simulink model "sdl_testbed"  (R2022b)
settings: Solver=VariableStepAuto  StartTime=0.0  StopTime=5  RelTol=1e-3  AbsTol=1e-3  EnableMultiTasking=on
PreLoadFcn:
  | MFormulaCoeff.DryTarmac = [10 1.9 1 0.97];
  | MFormulaCoeff.WetTarmac = [12 2.3 0.82 1];
  | MFormulaCoeff.Snow         = [5 2 0.3 1];
  | MFormulaCoeff.Ice            = [4 2 0.1 1];
libraries: sdl_lib x22, nesl_utility x9, fl_ps_legacy_lib x5, fl_lib x4, simulink x1
(part 2 of 3)

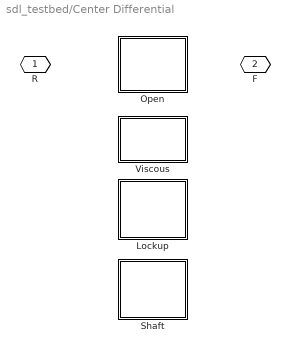
== system sdl_testbed/Center Differential ==
  Lockup : Subsystem  Tag=PublishSubsystem  VariantControl=Lockup
      mask Display:
      | %patch([0;227.23643342033;227.23643342033;0;0;0.472425017505884;0.472425017505884;226.764008402824;226.764008402824;0.472425017505884;0], [170.545431319624;170.545431319624;0;0;170.545431319624;170.073006302118;0.472425017505884;0.472425017505884;170.073006302118;170.073006302118;170.545431319624], [1;1;1])
      | plot([0;227.23643342033;227.23643342033;0;0;0.472425017505884;0.472425017505884;226.764008402824;226.764008402824;0.472425017505884;0], [170.545431319624;170.545431319624;0;0;170.545431319624;170.073006302118;0.472425017505884;0.472425017505884;170.073006302118;170.073006302118;170.545431319624])
      | plot([136.294617550448;187.000220911577], [85.2727156598121;85.2727156598121])
      | plot([40.236212508752942;90.9418158698827], [85.2727156598121;85.2727156598121])
      | patch([130.625517340377;136.294617550448;136.294617550448;130.625517340377;130.625517340377], [141.963717760518;141.963717760518;28.581713559106;28.581713559106;141.963717760518], [0;0;0])
      | plot([130.625517340377;136.294617550448;136.294617550448;130.625517340377;130.625517340377], [141.963717760518;141.963717760518;28.581713559106;28.581713559106;141.963717760518])
      | patch([90.9418158698827;96.6109160799533;96.6109160799533;90.9418158698827;90.9418158698827], [141.963717760518;141.963717760518;28.581713559106;28.581713559106;141.963717760518], [0;0;0])
      | plot([90.9418158698827;96.6109160799533;96.6109160799533;90.9418158698827;90.9418158698827], [141.963717760518;141.963717760518;28.581713559106;28.581713559106;141.963717760518])
      | patch([110.78366660513;116.4527668152;116.4527668152;110.78366660513;110.78366660513], [141.963717760518;141.963717760518;28.581713559106;28.581713559106;141.963717760518], [0;0;0])
      | plot([110.78366660513;116.4527668152;116.4527668152;110.78366660513;110.78366660513], [141.963717760518;141.963717760518;28.581713559106;28.581713559106;141.963717760518])
  Open : Subsystem  VariantControl=Open
      mask Display:
      | %patch([0;227.23643342033;227.23643342033;0;0;0.472425017505884;0.472425017505884;226.764008402824;226.764008402824;0.472425017505884;0], [170.545431319624;170.545431319624;0;0;170.545431319624;170.073006302118;0.472425017505884;0.472425017505884;170.073006302118;170.073006302118;170.545431319624], [1;1;1])
      | plot([0;227.23643342033;227.23643342033;0;0;0.472425017505884;0.472425017505884;226.764008402824;226.764008402824;0.472425017505884;0], [170.545431319624;170.545431319624;0;0;170.545431319624;170.073006302118;0.472425017505884;0.472425017505884;170.073006302118;170.073006302118;170.545431319624])
      | plot([136.294617550448;187.000220911577], [85.2727156598121;85.2727156598121])
      | plot([40.236212508752942;90.9418158698827], [85.2727156598121;85.2727156598121])
  Shaft : Subsystem  VariantControl=Shaft
      mask Display:
      | %patch([0;227.23643342033;227.23643342033;0;0;0.472425017505884;0.472425017505884;226.764008402824;226.764008402824;0.472425017505884;0], [170.545431319624;170.545431319624;0;0;170.545431319624;170.073006302118;0.472425017505884;0.472425017505884;170.073006302118;170.073006302118;170.545431319624], [1;1;1])
      | plot([0;227.23643342033;227.23643342033;0;0;0.472425017505884;0.472425017505884;226.764008402824;226.764008402824;0.472425017505884;0], [170.545431319624;170.545431319624;0;0;170.545431319624;170.073006302118;0.472425017505884;0.472425017505884;170.073006302118;170.073006302118;170.545431319624])
      | patch([40.236212508752942;40.236212508752942;187.9418158698827;187.9418158698827;40.236212508752942], [80.2727156598121;90.2727156598121;90.2727156598121;80.2727156598121;80.2727156598121])
  Viscous : Subsystem  VariantControl=Viscous
      mask Display:
      | %patch([-40;267.23643342033;267.23643342033;-40;-40;-40.472425017505884;-40.472425017505884;266.764008402824;266.764008402824;-40.472425017505884;-40], [170.545431319624;170.545431319624;0;0;170.545431319624;170.073006302118;0.472425017505884;0.472425017505884;170.073006302118;170.073006302118;170.545431319624], [1;1;1])
      | plot([-40;267.23643342033;267.23643342033;-40;-40;-40.472425017505884;-40.472425017505884;266.764008402824;266.764008402824;-40.472425017505884;-40], [170.545431319624;170.545431319624;0;0;170.545431319624;170.073006302118;0.472425017505884;0.472425017505884;170.073006302118;170.073006302118;170.545431319624])
      | plot([15.236212508752942;113.618216710165], [85.2727156598121;85.2727156598121])
      | plot([71.0999651346356;156.136468285695;156.136468285695;71.0999651346356], [144.798267865554;122.121867025271;48.4235642943531;25.7471634540707])
      | plot([156.136468285695;212.000220911577], [85.2727156598121;85.2727156598121])
      | plot([113.618216710165;113.618216710165], [123.570637078956;46.4078842196614])
      | plot([113.618216710165;113.618216710165], [46.4078842196614;45.5890141893178])
      | plot([96.6109160799533;136.294617550448], [42.7544640842825;51.2581143993884])
      | plot([93.776365974918;133.460067445412], [127.790967235342;119.287316920236])
  R : PMIOPort  Side=Left
  F : PMIOPort  Port=2  Side=Right

== system sdl_testbed/Front Differential ==
  Open : Subsystem  VariantControl=Open
      mask Display:
      | plot([73.6983027309179;73.6983027309179], [209.756707772613;130.389304831624])
      | plot([73.6983027309179;39.6837014704943], [170.073006302118;170.073006302118])
      | plot([62.3601023107767;85.0365031510592], [221.094908192754;198.418507352471])
      | plot([85.0365031510592;62.3601023107767], [141.727505251765;119.051104411483])
      | plot([102.043803781271;119.051104411483;119.051104411483;198.418507352471;198.418507352471], [181.41120672226;181.41120672226;260.778609663248;260.778609663248;277.78591029346])
      | plot([164.403906092048;255.109509453177], [226.764008402824;226.764008402824])
      | plot([153.065705671906;153.065705671906], [215.425807982683;124.720204621553])
      | plot([209.756707772613;209.756707772613], [317.469611763954;226.764008402824])
      | plot([187.08030693233;198.418507352471], [277.78591029346;277.78591029346])
      | plot([141.727505251765;164.403906092048], [226.764008402824;204.087607562542])
      | plot([175.742106512189;153.065705671906], [124.720204621553;102.043803781271])
      | plot([153.065705671906;175.742106512189], [238.102208822966;215.425807982683])
      | plot([209.756707772613;209.756707772613], [113.382004201412;22.6764008402824])
      | plot([164.403906092048;141.727505251765], [136.058405041695;113.382004201412])
      | plot([243.771309033036;266.447709873319], [124.720204621553;102.043803781271])
      | plot([266.447709873319;243.771309033036], [238.102208822966;215.425807982683])
      | plot([164.403906092048;255.109509453177], [113.382004201412;113.382004201412])
      | plot([187.08030693233;198.418507352471;198.418507352471;119.051104411483;119.051104411483;102.043803781271;102.043803781271], [62.3601023107767;62.3601023107767;79.3674029409885;79.3674029409885;158.734805881977;158.734805881977;147.396605461836])
      | plot([102.043803781271;153.065705671906], [170.073006302118;170.073006302118])
      | plot([102.043803781271;102.043803781271], [181.41120672226;192.749407142401])
      | plot([96.3747035712004;73.6983027309179], [130.389304831624;107.712903991342])
      | plot([85.0365031510592;119.051104411483], [119.051104411483;119.051104411483])
      | plot([-20;-20;360.146012604237;360.146012604237;-20], [360.146012604237;-20;-20;360.146012604237;360.146012604237])
  Torsen : Subsystem  VariantControl=Torsen
      mask Display:
      | plot([73.6983027309179;73.6983027309179], [209.756707772613;130.389304831624])
      | plot([73.6983027309179;39.6837014704943], [170.073006302118;170.073006302118])
      | 
      | % Planet Gear
      | plot([164.403906092048;255.109509453177;255.109509453177;164.403906092048;164.403906092048], [226.764008402824;226.764008402824;226.764008402824-50;226.764008402824-50;226.764008402824])
      | plot([164.403906092048;255.109509453177;255.109509453177;164.403906092048;164.403906092048], [113.382004201412;113.382004201412;113.382004201412+50;113.382004201412+50;113.382004201412])
      | plot([164.403906092048  ;164.403906092048+50]+ 0, [176.764008402824   ;176.764008402824+50])
      | plot([164.403906092048  ;164.403906092048+50]+20, [176.764008402824   ;176.764008402824+50])
      | plot([164.403906092048  ;164.403906092048+50]+40, [176.764008402824   ;176.764008402824+50])
      | plot([164.403906092048  ;164.403906092048+30]+60, [176.764008402824   ;176.764008402824+30])
      | plot([164.403906092048+20;164.403906092048+50]-20,[176.764008402824+20;176.764008402824+50])
      | 
      | plot([164.403906092048  ;164.403906092048+50]+ 0, [113.382004201412   ;113.382004201412+50])
      | plot([164.403906092048  ;164.403906092048+50]+20, [113.382004201412   ;113.382004201412+50])
      | plot([164.403906092048  ;164.403906092048+50]+40, [113.382004201412   ;113.382004201412+50])
      | plot([164.403906092048  ;164.403906092048+30]+60, [113.382004201412   ;113.382004201412+30])
      | plot([164.403906092048+20;164.403906092048+50]-20,[113.382004201412+20;113.382004201412+50])
      | 
      | plot(sin(0:0.1:6*pi)*20+140,cos(0:0.1:6*pi)*25+138);
      | plot(sin(0:0.1:6*pi)*25+140,cos(0:0.1:6*pi)*32+138);
      | plot(sin(0:0.1:6*pi)*20+140,cos(0:0.1:6*pi)*25+203);
      | plot(sin(0:0.1:6*pi)*25+140,cos(0:0.1:6*pi)*32+203);
      | 
      | 
      | plot([209.756707772613;209.756707772613], [317.469611763954;226.764008402824])
      | plot([209.756707772613;209.756707772613], [113.382004201412;22.6764008402824])
      | 
      | % Housing
      | plot([102.043803781271;119.051104411483;119.051104411483;198.418507352471;198.418507352471]-28, [181.41120672226;181.41120672226;260.778609663248;260.778609663248;277.78591029346])
      | plot([102.043803781271;102.043803781271]-28, [181.41120672226;192.749407142401])
      | plot([187.08030693233;198.418507352471]-28, [277.78591029346;277.78591029346])
      | plot([187.08030693233;198.418507352471;198.418507352471;119.051104411483;119.051104411483;102.043803781271;102.043803781271]-28, [62.3601023107767;62.3601023107767;79.3674029409885;79.3674029409885;158.734805881977;158.734805881977;147.396605461836])
      | 
      | plot([-20;-20;330.146012604237;330.146012604237;-20], [370.146012604237;-20;-20;370.146012604237;370.146012604237])
  D : PMIOPort  Side=Left
  S1 : PMIOPort  Port=2  Side=Right
  S2 : PMIOPort  Port=3  Side=Right

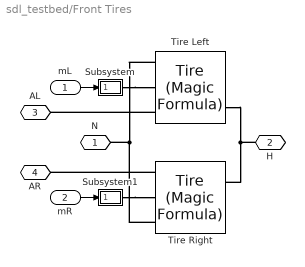
== system sdl_testbed/Front Tires ==
  mL : Inport
  mR : Inport  Port=2
  Subsystem : Subsystem
      mask Display: disp('PS')
  Subsystem1 : Subsystem
      mask Display: disp('PS')
  Tire Left : sdl_lib/Tires & Vehicles/Tire (Magic Formula)  parameterization=4  F_z1=3e+3 N  F_x1=3.5e+3 N  kappa1=10  B_m=10  C_m=1.9  D_m=1  E_m=0.97  fz0=4e+3 N  p_Cx=1.685  p_Dx=[ 1.21 -0.037 ]  p_Ex=[ 0.344 0.095 -0.02 0 ]  p_Kx=[ 21.51 -0.163 0.245 ]  p_Hx=[ -0.002 0.002 ]  p_Vx=[ 0 0 ]  r_e=0.3 m  model_compliance=0  stiffness=1e+6 N/m  damping=1000 N/(m/s)  model_inertia=1  inertia=1 kg*m^2  initial_velocity=0 rad/s  model_resistance=0  resistance_model=1  coeff=0.015  p_tire=250e3 Pa  alpha=-0.003  beta=0.97  coeff_a=84e-4  coeff_b=6.2e-4 s/m  coeff_c=1.6e-4 s^2/m^2  v_thr=1e-3 m/s  v_tr_thr=0.1 m/s
      settings: InternalSimscapePortConfiguration="{\"Bottom\":[],\"Left\":[{\"id\":\"N\",\"label\":\"N\",\"type\":\"input\"},{\"id\":\"M\",\"label\":\"M\",\"type\":\"input\"},{\"id\":\"A\",\"label\":\"A\",\"type\":\"foundation.mechanical.rotational.rotational\"}],\"Right\":[{\"id\":\"S\",\"label\":\"S\",\"type\":\"output\"},{\"id\":\"H\",\"label\":\"H\",\"type\":\"foundation.mechanical.translational.translational\"}],\"Top\":[]}"
  Tire Right : sdl_lib/Tires & Vehicles/Tire (Magic Formula)  parameterization=4  F_z1=3e+3 N  F_x1=3.5e+3 N  kappa1=10  B_m=10  C_m=1.9  D_m=1  E_m=0.97  fz0=4e+3 N  p_Cx=1.685  p_Dx=[ 1.21 -0.037 ]  p_Ex=[ 0.344 0.095 -0.02 0 ]  p_Kx=[ 21.51 -0.163 0.245 ]  p_Hx=[ -0.002 0.002 ]  p_Vx=[ 0 0 ]  r_e=0.3 m  model_compliance=0  stiffness=1e+6 N/m  damping=1000 N/(m/s)  model_inertia=1  inertia=1 kg*m^2  initial_velocity=0 rad/s  model_resistance=0  resistance_model=1  coeff=0.015  p_tire=250e3 Pa  alpha=-0.003  beta=0.97  coeff_a=84e-4  coeff_b=6.2e-4 s/m  coeff_c=1.6e-4 s^2/m^2  v_thr=1e-3 m/s  v_tr_thr=0.1 m/s
      settings: InternalSimscapePortConfiguration="{\"Bottom\":[],\"Left\":[{\"id\":\"N\",\"label\":\"N\",\"type\":\"input\"},{\"id\":\"M\",\"label\":\"M\",\"type\":\"input\"},{\"id\":\"A\",\"label\":\"A\",\"type\":\"foundation.mechanical.rotational.rotational\"}],\"Right\":[{\"id\":\"S\",\"label\":\"S\",\"type\":\"output\"},{\"id\":\"H\",\"label\":\"H\",\"type\":\"foundation.mechanical.translational.translational\"}],\"Top\":[]}"
  N : PMIOPort  Side=Right
  H : PMIOPort  Port=2  Side=Right
  AL : PMIOPort  Port=3  Side=Right
  AR : PMIOPort  Port=4  Side=Right
  wires:
  mR/1 -> Subsystem1/1(In1)
  mL/1 -> Subsystem/1(In1)
  connections:
  Subsystem/RConn1 -- Tire Left/LConn2
  Subsystem1/RConn1 -- Tire Right/LConn2
  Tire Right/LConn3 -- AR/RConn1
  Tire Left/LConn1 -- Tire Right/LConn1 -- N/RConn1
  Tire Left/RConn2 -- Tire Right/RConn2 -- H/RConn1
  Tire Left/LConn3 -- AL/RConn1

== system sdl_testbed/Rear Differential ==
  Open : Subsystem  Tag=PublishSubsystem  VariantControl=Open
      mask Display:
      | plot([73.6983027309179;73.6983027309179], [209.756707772613;130.389304831624])
      | plot([73.6983027309179;39.6837014704943], [170.073006302118;170.073006302118])
      | plot([62.3601023107767;85.0365031510592], [221.094908192754;198.418507352471])
      | plot([85.0365031510592;62.3601023107767], [141.727505251765;119.051104411483])
      | plot([102.043803781271;119.051104411483;119.051104411483;198.418507352471;198.418507352471], [181.41120672226;181.41120672226;260.778609663248;260.778609663248;277.78591029346])
      | plot([164.403906092048;255.109509453177], [226.764008402824;226.764008402824])
      | plot([153.065705671906;153.065705671906], [215.425807982683;124.720204621553])
      | plot([209.756707772613;209.756707772613], [317.469611763954;226.764008402824])
      | plot([187.08030693233;198.418507352471], [277.78591029346;277.78591029346])
      | plot([141.727505251765;164.403906092048], [226.764008402824;204.087607562542])
      | plot([175.742106512189;153.065705671906], [124.720204621553;102.043803781271])
      | plot([153.065705671906;175.742106512189], [238.102208822966;215.425807982683])
      | plot([209.756707772613;209.756707772613], [113.382004201412;22.6764008402824])
      | plot([164.403906092048;141.727505251765], [136.058405041695;113.382004201412])
      | plot([243.771309033036;266.447709873319], [124.720204621553;102.043803781271])
      | plot([266.447709873319;243.771309033036], [238.102208822966;215.425807982683])
      | plot([164.403906092048;255.109509453177], [113.382004201412;113.382004201412])
      | plot([187.08030693233;198.418507352471;198.418507352471;119.051104411483;119.051104411483;102.043803781271;102.043803781271], [62.3601023107767;62.3601023107767;79.3674029409885;79.3674029409885;158.734805881977;158.734805881977;147.396605461836])
      | plot([102.043803781271;153.065705671906], [170.073006302118;170.073006302118])
      | plot([102.043803781271;102.043803781271], [181.41120672226;192.749407142401])
      | plot([96.3747035712004;73.6983027309179], [130.389304831624;107.712903991342])
      | plot([85.0365031510592;119.051104411483], [119.051104411483;119.051104411483])
      | plot([-20;-20;360.146012604237;360.146012604237;-20], [360.146012604237;-20;-20;360.146012604237;360.146012604237])
  Torsen : Subsystem  Tag=PublishSubsystem  VariantControl=Torsen
      mask Display:
      | plot([73.6983027309179;73.6983027309179], [209.756707772613;130.389304831624])
      | plot([73.6983027309179;39.6837014704943], [170.073006302118;170.073006302118])
      | 
      | % Planet Gear
      | plot([164.403906092048;255.109509453177;255.109509453177;164.403906092048;164.403906092048], [226.764008402824;226.764008402824;226.764008402824-50;226.764008402824-50;226.764008402824])
      | plot([164.403906092048;255.109509453177;255.109509453177;164.403906092048;164.403906092048], [113.382004201412;113.382004201412;113.382004201412+50;113.382004201412+50;113.382004201412])
      | plot([164.403906092048  ;164.403906092048+50]+ 0, [176.764008402824   ;176.764008402824+50])
      | plot([164.403906092048  ;164.403906092048+50]+20, [176.764008402824   ;176.764008402824+50])
      | plot([164.403906092048  ;164.403906092048+50]+40, [176.764008402824   ;176.764008402824+50])
      | plot([164.403906092048  ;164.403906092048+30]+60, [176.764008402824   ;176.764008402824+30])
      | plot([164.403906092048+20;164.403906092048+50]-20,[176.764008402824+20;176.764008402824+50])
      | 
      | plot([164.403906092048  ;164.403906092048+50]+ 0, [113.382004201412   ;113.382004201412+50])
      | plot([164.403906092048  ;164.403906092048+50]+20, [113.382004201412   ;113.382004201412+50])
      | plot([164.403906092048  ;164.403906092048+50]+40, [113.382004201412   ;113.382004201412+50])
      | plot([164.403906092048  ;164.403906092048+30]+60, [113.382004201412   ;113.382004201412+30])
      | plot([164.403906092048+20;164.403906092048+50]-20,[113.382004201412+20;113.382004201412+50])
      | 
      | plot(sin(0:0.1:6*pi)*20+140,cos(0:0.1:6*pi)*25+138);
      | plot(sin(0:0.1:6*pi)*25+140,cos(0:0.1:6*pi)*32+138);
      | plot(sin(0:0.1:6*pi)*20+140,cos(0:0.1:6*pi)*25+203);
      | plot(sin(0:0.1:6*pi)*25+140,cos(0:0.1:6*pi)*32+203);
      | 
      | 
      | plot([209.756707772613;209.756707772613], [317.469611763954;226.764008402824])
      | plot([209.756707772613;209.756707772613], [113.382004201412;22.6764008402824])
      | 
      | % Housing
      | plot([102.043803781271;119.051104411483;119.051104411483;198.418507352471;198.418507352471]-28, [181.41120672226;181.41120672226;260.778609663248;260.778609663248;277.78591029346])
      | plot([102.043803781271;102.043803781271]-28, [181.41120672226;192.749407142401])
      | plot([187.08030693233;198.418507352471]-28, [277.78591029346;277.78591029346])
      | plot([187.08030693233;198.418507352471;198.418507352471;119.051104411483;119.051104411483;102.043803781271;102.043803781271]-28, [62.3601023107767;62.3601023107767;79.3674029409885;79.3674029409885;158.734805881977;158.734805881977;147.396605461836])
      | 
      | plot([-20;-20;330.146012604237;330.146012604237;-20], [370.146012604237;-20;-20;370.146012604237;370.146012604237])
  D : PMIOPort  Side=Left
  S1 : PMIOPort  Port=2  Side=Right
  S2 : PMIOPort  Port=3  Side=Right

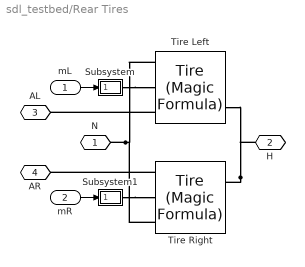
== system sdl_testbed/Rear Tires ==
  mL : Inport
  mR : Inport  Port=2
  Subsystem : Subsystem
      mask Display: disp('PS')
  Subsystem1 : Subsystem
      mask Display: disp('PS')
  Tire Left : sdl_lib/Tires & Vehicles/Tire (Magic Formula)  parameterization=4  F_z1=3e+3 N  F_x1=3.5e+3 N  kappa1=10  B_m=10  C_m=1.9  D_m=1  E_m=0.97  fz0=4e+3 N  p_Cx=1.685  p_Dx=[ 1.21 -0.037 ]  p_Ex=[ 0.344 0.095 -0.02 0 ]  p_Kx=[ 21.51 -0.163 0.245 ]  p_Hx=[ -0.002 0.002 ]  p_Vx=[ 0 0 ]  r_e=0.3 m  model_compliance=0  stiffness=1e+6 N/m  damping=1000 N/(m/s)  model_inertia=1  inertia=1 kg*m^2  initial_velocity=0 rad/s  model_resistance=0  resistance_model=1  coeff=0.015  p_tire=250e3 Pa  alpha=-0.003  beta=0.97  coeff_a=84e-4  coeff_b=6.2e-4 s/m  coeff_c=1.6e-4 s^2/m^2  v_thr=1e-3 m/s  v_tr_thr=0.1 m/s
      settings: InternalSimscapePortConfiguration="{\"Bottom\":[],\"Left\":[{\"id\":\"N\",\"label\":\"N\",\"type\":\"input\"},{\"id\":\"M\",\"label\":\"M\",\"type\":\"input\"},{\"id\":\"A\",\"label\":\"A\",\"type\":\"foundation.mechanical.rotational.rotational\"}],\"Right\":[{\"id\":\"S\",\"label\":\"S\",\"type\":\"output\"},{\"id\":\"H\",\"label\":\"H\",\"type\":\"foundation.mechanical.translational.translational\"}],\"Top\":[]}"
  Tire Right : sdl_lib/Tires & Vehicles/Tire (Magic Formula)  parameterization=4  F_z1=3e+3 N  F_x1=3.5e+3 N  kappa1=10  B_m=10  C_m=1.9  D_m=1  E_m=0.97  fz0=4e+3 N  p_Cx=1.685  p_Dx=[ 1.21 -0.037 ]  p_Ex=[ 0.344 0.095 -0.02 0 ]  p_Kx=[ 21.51 -0.163 0.245 ]  p_Hx=[ -0.002 0.002 ]  p_Vx=[ 0 0 ]  r_e=0.3 m  model_compliance=0  stiffness=1e+6 N/m  damping=1000 N/(m/s)  model_inertia=1  inertia=1 kg*m^2  initial_velocity=0 rad/s  model_resistance=0  resistance_model=1  coeff=0.015  p_tire=250e3 Pa  alpha=-0.003  beta=0.97  coeff_a=84e-4  coeff_b=6.2e-4 s/m  coeff_c=1.6e-4 s^2/m^2  v_thr=1e-3 m/s  v_tr_thr=0.1 m/s
      settings: InternalSimscapePortConfiguration="{\"Bottom\":[],\"Left\":[{\"id\":\"N\",\"label\":\"N\",\"type\":\"input\"},{\"id\":\"M\",\"label\":\"M\",\"type\":\"input\"},{\"id\":\"A\",\"label\":\"A\",\"type\":\"foundation.mechanical.rotational.rotational\"}],\"Right\":[{\"id\":\"S\",\"label\":\"S\",\"type\":\"output\"},{\"id\":\"H\",\"label\":\"H\",\"type\":\"foundation.mechanical.translational.translational\"}],\"Top\":[]}"
  N : PMIOPort  Side=Right
  H : PMIOPort  Port=2  Side=Right
  AL : PMIOPort  Port=3  Side=Right
  AR : PMIOPort  Port=4  Side=Right
  wires:
  mL/1 -> Subsystem/1(In1)
  mR/1 -> Subsystem1/1(In1)
  connections:
  Tire Left/LConn3 -- AL/RConn1
  Tire Right/RConn2 -- H/RConn1 -- Tire Left/RConn2
  N/RConn1 -- Tire Right/LConn1 -- Tire Left/LConn1
  Tire Right/LConn3 -- AR/RConn1
  Subsystem1/RConn1 -- Tire Right/LConn2
  Subsystem/RConn1 -- Tire Left/LConn2

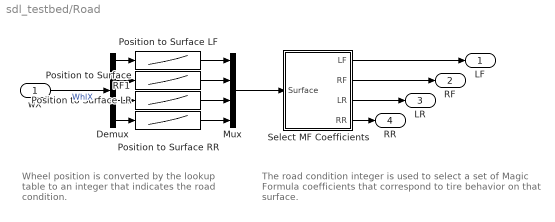
== system sdl_testbed/Road ==
  note: Wheel position is converted by the
      | lookup table to an integer
      | that indicates the road condition.
  note: The road condition integer is used to select
      | a set of Magic Formula coefficients
      | that correspond to tire behavior on that surface.
  wX : Inport
  Demux : Demux
  Mux : Mux
  Position to Surface LF : Lookup_n-D  NumberOfTableDimensions=1  LookupTableObject=''  BreakpointsForDimension1=surface_xpos  BeginIndexSearchUsingPreviousIndexResult=on  Table=surface_LF  InterpMethod=Flat  InternalRulePriority=Speed  RndMeth=Simplest
  Position to Surface LR : Lookup_n-D  NumberOfTableDimensions=1  LookupTableObject=''  BreakpointsForDimension1=surface_xpos  BeginIndexSearchUsingPreviousIndexResult=on  Table=surface_LR  InterpMethod=Flat  InternalRulePriority=Speed  RndMeth=Simplest
  Position to Surface RF1 : Lookup_n-D  NumberOfTableDimensions=1  LookupTableObject=''  BreakpointsForDimension1=surface_xpos  BeginIndexSearchUsingPreviousIndexResult=on  Table=surface_RF  InterpMethod=Flat  InternalRulePriority=Speed  RndMeth=Simplest
  Position to Surface RR : Lookup_n-D  NumberOfTableDimensions=1  LookupTableObject=''  BreakpointsForDimension1=surface_xpos  BeginIndexSearchUsingPreviousIndexResult=on  Table=surface_RR  InterpMethod=Flat  InternalRulePriority=Speed  RndMeth=Simplest
  Select MF Coefficients : Subsystem
  LF : Outport  VectorParamsAs1DForOutWhenUnconnected=off
  RF : Outport  Port=2  VectorParamsAs1DForOutWhenUnconnected=off
  LR : Outport  Port=3  VectorParamsAs1DForOutWhenUnconnected=off
  RR : Outport  Port=4  VectorParamsAs1DForOutWhenUnconnected=off
  wires:
  Select MF Coefficients/3(LR) -> LR/1
  Select MF Coefficients/4(RR) -> RR/1
  Select MF Coefficients/1(LF) -> LF/1
  Select MF Coefficients/2(RF) -> RF/1
  wX/1 -> Demux/1  "WhlX"
  Mux/1 -> Select MF Coefficients/1(Surface)
  Demux/1 -> Position to Surface LF/1
  Position to Surface LF/1 -> Mux/1
  Position to Surface RR/1 -> Mux/4
  Demux/4 -> Position to Surface RR/1
  Demux/2 -> Position to Surface RF1/1
  Position to Surface RF1/1 -> Mux/2
  Position to Surface LR/1 -> Mux/3
  Demux/3 -> Position to Surface LR/1

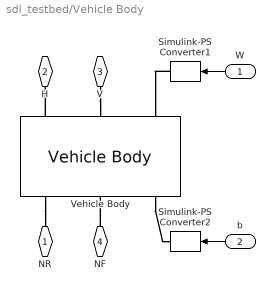
== system sdl_testbed/Vehicle Body ==
  W : Inport
  b : Inport  Port=2
  Simulink-PS Converter1 : nesl_utility/Simulink-PS Converter  PhysicalDomain=network_engine_domain  SubClassName=ps_input  LeftPortType=input  RightPortType=output  PseudoPeriodic=off  Frequencies=[]  NoiseDistribution=none  NoiseParameters=[]  Unit=m/s  AffineConversion=off  FilteringAndDerivatives=zero  SimscapeFilterOrder=1  InputFilterTimeConstant=.001  UdotUserProvided=1
  Simulink-PS Converter2 : nesl_utility/Simulink-PS Converter  PhysicalDomain=network_engine_domain  SubClassName=ps_input  LeftPortType=input  RightPortType=output  PseudoPeriodic=off  Frequencies=[]  NoiseDistribution=none  NoiseParameters=[]  Unit=deg  AffineConversion=off  FilteringAndDerivatives=zero  SimscapeFilterOrder=1  InputFilterTimeConstant=.001  UdotUserProvided=1
  Vehicle Body : sdl_lib/Tires & Vehicles/Vehicle Body  mass=1000 kg  n_w=2  x_f=1.4 m  x_r=1.6 m  y_c=0.5 m  mass_var=simscape.enum.onoff.off  g=9.81 m/s^2  liftoff_warning=0  area=3 m^2  Cd=0.4  rho=1.18 kg/m^3  model_pitch=0  inertia=4000 kg*m^2  suspension_model=1  k_f=1e4 N/m  b_f=1e4 N/(m/s)  k_r=1e4 N/m  b_r=1e4 N/(m/s)  k_f_TLU=[-2000, -1000, 0, 1000, 2000] N  x_f_TLU=[-.4, -.2, 0, .2, .4] m  b_f_TLU=[-200, -100, 0, 100, 200] N  v_f_TLU=[-4, -2, 0, 2, 4] m/s  k_r_TLU=[-2000, -1000, 0, 1000, 2000] N  x_r_TLU=[-.4, -.2, 0, .2, .4] m  b_r_TLU=[-200, -100, 0, 100, 200] N  v_r_TLU=[-4, -2, 0, 2, 4] m/s  interp_method=simscape.enum.interpolation.linear  extrap_method=simscape.enum.extrapolation.linear  model_hardstop=0  upper_bound_f=.25 m  lower_bound_f=-.25 m  stop_k_f=1e6 N/m  stop_b_f=150 N/(m/s)  upper_bound_r=.25 m  lower_bound_r=-.25 m  stop_k_r=1e6 N/m  stop_b_r=150 N/(m/s)  initial_pitch=0 rad  initial_pitch_rate=0 rad/s  v_specify=on  v_priority=High  v=0 m/s  v_nominal_specify=off  v_nominal_unit=m/s  v_nominal_value=1
  NR : PMIOPort  Side=Right
  H : PMIOPort  Port=2  Side=Right
  V : PMIOPort  Port=3  Side=Left
  NF : PMIOPort  Port=4  Side=Right
  wires:
  W/1 -> Simulink-PS Converter1/1
  b/1 -> Simulink-PS Converter2/1
  connections:
  Simulink-PS Converter1/RConn1 -- Vehicle Body/LConn3
  Vehicle Body/LConn1 -- H/RConn1
  Vehicle Body/RConn3 -- Simulink-PS Converter2/RConn1
  NF/RConn1 -- Vehicle Body/RConn2
  V/RConn1 -- Vehicle Body/LConn2
  Vehicle Body/RConn1 -- NR/RConn1

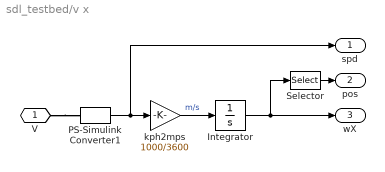
== system sdl_testbed/v x ==
  Integrator : Integrator  InitialCondition=[3 3 0 0]
  PS-Simulink Converter1 : nesl_utility/PS-Simulink Converter  PhysicalDomain=network_engine_domain  SubClassName=ps_output  LeftPortType=input  RightPortType=output  PseudoPeriodic=off  Frequencies=[]  VectorFormat=1-D array  Unit=km/hr  AffineConversion=off
  Selector : Selector  InputPortWidth=4  IndexOptions=Index vector (dialog)  Indices=[3]  OutputSizes=1
  kph2mps : Gain  Gain=1000/3600
  V : PMIOPort  Side=Left
  spd : Outport  VectorParamsAs1DForOutWhenUnconnected=off
  pos : Outport  Port=2  VectorParamsAs1DForOutWhenUnconnected=off
  wX : Outport  Port=3  VectorParamsAs1DForOutWhenUnconnected=off
  wires:
  PS-Simulink Converter1/1 -> spd/1, kph2mps/1
  Integrator/1 -> wX/1, Selector/1
  kph2mps/1 -> Integrator/1  "m/s"
  Selector/1 -> pos/1
  connections:
  V/RConn1 -- PS-Simulink Converter1/LConn1

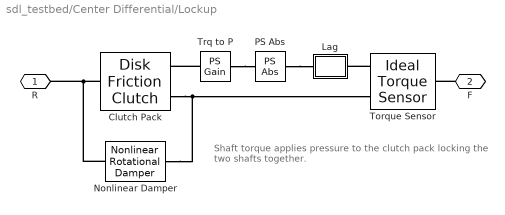
== system sdl_testbed/Center Differential/Lockup ==
  note: Shaft torque applies pressure to the clutch pack
      | locking the two shafts together.
  Clutch Pack : sdl_lib/Clutches/Disk Friction Clutch  geometry_model=1  r_eff=130 mm  d_o=150 mm  d_i=100 mm  nS=4  piston_area=0.001 m^2  unidirectional=0  friction_model=1  mu_w_vector=[ 0 0.1 0.2 0.3 0.4 0.5 1 2 5 10 100 1000 ] rad/s  temperature_TLU=[280.0, 300.0, 320.0] K  mu_static=0.35  mu_static_vector=[0.4, 0.38, 0.36]  mu_coulomb=0.3  mu_coulomb_vector=[ 0.29 0.28 0.26 0.22 0.21 0.2 0.2 0.19 0.19 0.19 0.19 0.19 ]  mu_coulomb_temp_vector=[0.3, 0.28, 0.25]  mu_coulomb_matrix=[0.34, 0.32, 0.3; 0.3, 0.28, 0.25; 0.25, 0.2, 0.15]  mu_interp_method=1  mu_extrap_method=1  d_f=1  w_tol=0.001 rad/s  pressure_min=100 Pa  mu_visc=0 N*m/(rad/s)  initial_state_locked=0  enable_faults=simscape.enum.onoff.off  fault_type=sdl.enum.clutchFault.lock  external_fault=simscape.enum.onoff.off  temporal_fault=simscape.enum.onoff.off  fault_time=5 s  report_fault=simscape.enum.assert.action.none  thermal_mass=25 kJ/K  T_init=300 K
      settings: InternalSimscapePortConfiguration="{\"Bottom\":[],\"Left\":[{\"id\":\"P\",\"label\":\"P\",\"type\":\"input\"},{\"id\":\"B\",\"label\":\"B\",\"type\":\"foundation.mechanical.rotational.rotational\"}],\"Right\":[{\"id\":\"F\",\"label\":\"F\",\"type\":\"foundation.mechanical.rotational.rotational\"}],\"Top\":[]}"
  Lag : Subsystem
  Nonlinear Damper : sdl_lib/Couplings & Drives/Springs & Dampers/Nonlinear Rotational Damper  parameterization=1  symmetry=1  coefficient_vector=[ 0 0 0 0 1e-4 ] N*m/(rad/s)  positive_coefficient_vector=[ 1e-4 0 1e-5 0 1e-6 ] N*m/(rad/s)  negative_coefficient_vector=[ 0.001 -1e-5 1e-4 0 0 ] N*m/(rad/s)  angular_velocity_vector=[ -1 -0.5 -0.3 -0.1 0.1 0.3 0.5 1 ] rad/s  torque_vector=[ -0.001 -4e-4 -2e-4 -5e-5 5e-5 2e-4 4e-4 0.001 ] N*m  interp_method=1  extrap_method=1
      settings: InternalSimscapePortConfiguration="{\"Bottom\":[],\"Left\":[{\"id\":\"R\",\"label\":\"R\",\"type\":\"foundation.mechanical.rotational.rotational\"}],\"Right\":[{\"id\":\"C\",\"label\":\"C\",\"type\":\"foundation.mechanical.rotational.rotational\"}],\"Top\":[]}"
  PS Abs : fl_ps_legacy_lib/Legacy Physical Signals/Nonlinear Operators/PS Abs
      settings: InternalSimscapePortConfiguration="{\"Bottom\":[],\"Left\":[{\"id\":\"I\",\"label\":\"\",\"type\":\"input\"}],\"Right\":[{\"id\":\"O\",\"label\":\"\",\"type\":\"output\"}],\"Top\":[]}"
  Torque Sensor : fl_lib/Mechanical/Mechanical Sensors/Ideal Torque Sensor
  Trq to P : fl_ps_legacy_lib/Legacy Physical Signals/Functions/PS Gain  gain=20000
  R : PMIOPort  Side=Left
  F : PMIOPort  Port=2  Side=Right
  connections:
  Clutch Pack/LConn2 -- Torque Sensor/RConn1 -- Nonlinear Damper/RConn1
  Clutch Pack/RConn1 -- R/RConn1 -- Nonlinear Damper/LConn1
  F/RConn1 -- Torque Sensor/LConn1
  Trq to P/LConn1 -- PS Abs/RConn1
  Torque Sensor/RConn2 -- Lag/LConn1
  Trq to P/RConn1 -- Clutch Pack/LConn1
  PS Abs/LConn1 -- Lag/RConn1

== system sdl_testbed/Center Differential/Open ==
  Damper : fl_lib/Mechanical/Rotational Elements/Rotational Damper  D=0 N*m/(rad/s)  w_specify=off  w_priority=None  w=0 rad/s  w_nominal_specify=off  w_nominal_unit=rad/s  w_nominal_value=1  t_specify=off  t_priority=None  t=0 N*m  t_nominal_specify=off  t_nominal_unit=N*m  t_nominal_value=1
      settings: AttributesFormatString=Damping = %<D>
  R : PMIOPort  Side=Left
  F : PMIOPort  Port=2  Side=Right
  connections:
  Damper/RConn1 -- F/RConn1
  Damper/LConn1 -- R/RConn1

== system sdl_testbed/Center Differential/Shaft ==
  Torsional Spring-Damper : sdl_lib/Couplings & Drives/Torsional Spring-Damper  k=10000 N*m/rad  mu_visc=1000 N*m/(rad/s)  trq_coulomb=0 N*m  static_kinetic_ratio=1.1  w_tol=0.001 rad/s  model_hardstop=0  upper_bound=10 deg  lower_bound=-10 deg  k_endstop=1e+6 N*m/rad  D_endstop=10 N*m/(rad/s)  hardstop_model=3  transition=0.001 rad  x0=0 deg
      settings: InternalSimscapePortConfiguration="{\"Bottom\":[],\"Left\":[{\"id\":\"R\",\"label\":\"R\",\"type\":\"foundation.mechanical.rotational.rotational\"}],\"Right\":[{\"id\":\"C\",\"label\":\"C\",\"type\":\"foundation.mechanical.rotational.rotational\"}],\"Top\":[]}"
  R : PMIOPort  Side=Left
  F : PMIOPort  Port=2  Side=Right
  connections:
  Torsional Spring-Damper/LConn1 -- R/RConn1
  F/RConn1 -- Torsional Spring-Damper/RConn1

== system sdl_testbed/Center Differential/Viscous ==
  Nonlinear Damper : sdl_lib/Couplings & Drives/Springs & Dampers/Nonlinear Rotational Damper  parameterization=1  symmetry=1  coefficient_vector=[ 0 0 0 0 1e-4 ] N*m/(rad/s)  positive_coefficient_vector=[ 1e-4 0 1e-5 0 1e-6 ] N*m/(rad/s)  negative_coefficient_vector=[ 0.001 -1e-5 1e-4 0 0 ] N*m/(rad/s)  angular_velocity_vector=[ -1 -0.5 -0.3 -0.1 0.1 0.3 0.5 1 ] rad/s  torque_vector=[ -0.001 -4e-4 -2e-4 -5e-5 5e-5 2e-4 4e-4 0.001 ] N*m  interp_method=1  extrap_method=1
      settings: InternalSimscapePortConfiguration="{\"Bottom\":[],\"Left\":[{\"id\":\"R\",\"label\":\"R\",\"type\":\"foundation.mechanical.rotational.rotational\"}],\"Right\":[{\"id\":\"C\",\"label\":\"C\",\"type\":\"foundation.mechanical.rotational.rotational\"}],\"Top\":[]}"
  R : PMIOPort  Side=Left
  F : PMIOPort  Port=2  Side=Right
  connections:
  Nonlinear Damper/LConn1 -- R/RConn1
  Nonlinear Damper/RConn1 -- F/RConn1

== system sdl_testbed/Front Differential/Open ==
  Differential : sdl_lib/Gears/Differential  driveshaft_location=2  cd_ratio=1.33  friction_model=1  efficiency=[ 0.9 0.92 ]  temperature_TLU=[ 280 300 320 ] K  efficiency_ss_TLU=[ 0.95 0.9 0.85 ]  efficiency_cd_TLU=[ 0.95 0.9 0.85 ]  pwr_thr=[ 0.001 0.001 ] W  mu_visc=[ 0 0 ] N*m/(rad/s)  model_inertia=0  carrier_inertia=0.001 kg*m^2  planet_inertia=0.001 kg*m^2  thermal_mass=50 J/K  T_init=300 K
  D : PMIOPort  Side=Left
  S1 : PMIOPort  Port=2  Side=Right
  S2 : PMIOPort  Port=3  Side=Right
  connections:
  S2/RConn1 -- Differential/RConn2
  S1/RConn1 -- Differential/RConn1
  D/RConn1 -- Differential/LConn1

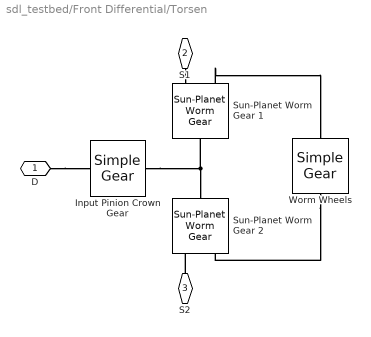
== system sdl_testbed/Front Differential/Torsen ==
  Input Pinion Crown Gear : sdl_lib/Gears/Simple Gear  ratio=2  rotation_direction=3-2*(1)  friction_model=1  T_noload=0.1 N*m  T_nom=5 N*m  efficiency_nom=0.8  efficiency=0.92  temperature_TLU=[ 280 300 320 ] K  load_TLU=[ 1 5 10 ] N*m  efficiency_TLU=[ 0.95 0.9 0.85 ]  efficiency_TLU2=[ 0.85 0.8 0.75; 0.95 0.9 0.85; 0.85 0.8 0.7 ]  w_thr=0.01 rad/s  pwr_thr=0.001 W  backlash_model=sdl.enum.backlashModel.Off  backlash_distance=1e-3 mm  x0=0 mm  r_base=0.1 m  hardstop_model=simscape.enum.hardstop.smooth  transition=1e-4 mm  backlash_stiffness=1e7 N/m  backlash_damping=1e6 N*s/m  e=0  v_tol=0.001 m/s  mu_visc=[ 0 0 ] N*m/(rad/s)  enable_faults=simscape.enum.onoff.off  efficiency_fault=0.05  external_fault=simscape.enum.onoff.off  temporal_fault=simscape.enum.onoff.off  fault_time=5 s  fault_angles=pi / 12 rad  report_fault=(1)-1  thermal_mass=50 J/K  temperature_specify=off  temperature_priority=High  temperature=300 K  temperature_nominal_specify=off  temperature_nominal_unit=K  temperature_nominal_value=1  x_backlash_specify=off  x_backlash_priority=None  x_backlash=0 mm  x_backlash_nominal_specify=off  x_backlash_nominal_unit=mm  x_backlash_nominal_value=1  f_hardstop_specify=off  f_hardstop_priority=None  f_hardstop=0 N  f_hardstop_nominal_specify=off  f_hardstop_nominal_unit=N  f_hardstop_nominal_value=1  v_backlash_specify=off  v_backlash_priority=None  v_backlash=0 m/s  v_backlash_nominal_specify=off  v_backlash_nominal_unit=m/s  v_backlash_nominal_value=1
  Sun-Planet Worm Gear 1 : sdl_lib/Gears/Planetary Subcomponents/Sun-Planet Worm Gear  ratio=2  thread_type=1  friction_model=2  friction_parameterization=2  pr_ang=17.5 deg  lead_ang=20 deg  fr_coeff=0.08  eff_wg=0.74  eff_gw=-0.1  temperature_TLU=[ 280 300 320 ] K  efficiency_wg_TLU=[ 0.75 0.7 0.65 ]  efficiency_gw_TLU=[ 0.5 0.45 0.4 ]  pwr_thr=0.001 W  mu_visc=[ 0 0 ] N*m/(rad/s)  thermal_mass=50 J/K  temperature_specify=off  temperature_priority=High  temperature=300 K  temperature_nominal_specify=off  temperature_nominal_unit=K  temperature_nominal_value=1
      settings: InternalSimscapePortConfiguration="{\"Bottom\":[],\"Left\":[{\"id\":\"C\",\"label\":\"C\",\"type\":\"foundation.mechanical.rotational.rotational\"}],\"Right\":[{\"id\":\"W\",\"label\":\"W\",\"type\":\"foundation.mechanical.rotational.rotational\"},{\"id\":\"S\",\"label\":\"S\",\"type\":\"foundation.mechanical.rotational.rotational\"}],\"Top\":[]}"
  Sun-Planet Worm Gear 2 : sdl_lib/Gears/Planetary Subcomponents/Sun-Planet Worm Gear  ratio=2  thread_type=1  friction_model=2  friction_parameterization=2  pr_ang=17.5 deg  lead_ang=20 deg  fr_coeff=0.08  eff_wg=0.74  eff_gw=-0.1  temperature_TLU=[ 280 300 320 ] K  efficiency_wg_TLU=[ 0.75 0.7 0.65 ]  efficiency_gw_TLU=[ 0.5 0.45 0.4 ]  pwr_thr=0.001 W  mu_visc=[ 0 0 ] N*m/(rad/s)  thermal_mass=50 J/K  temperature_specify=off  temperature_priority=High  temperature=300 K  temperature_nominal_specify=off  temperature_nominal_unit=K  temperature_nominal_value=1
      settings: InternalSimscapePortConfiguration="{\"Bottom\":[],\"Left\":[{\"id\":\"C\",\"label\":\"C\",\"type\":\"foundation.mechanical.rotational.rotational\"}],\"Right\":[{\"id\":\"W\",\"label\":\"W\",\"type\":\"foundation.mechanical.rotational.rotational\"},{\"id\":\"S\",\"label\":\"S\",\"type\":\"foundation.mechanical.rotational.rotational\"}],\"Top\":[]}"
  Worm Wheels : sdl_lib/Gears/Simple Gear  ratio=1  rotation_direction=3-2*(2)  friction_model=1  T_noload=0.1 N*m  T_nom=5 N*m  efficiency_nom=0.8  efficiency=0.92  temperature_TLU=[ 280 300 320 ] K  load_TLU=[ 1 5 10 ] N*m  efficiency_TLU=[ 0.95 0.9 0.85 ]  efficiency_TLU2=[ 0.85 0.8 0.75; 0.95 0.9 0.85; 0.85 0.8 0.7 ]  w_thr=0.01 rad/s  pwr_thr=0.001 W  backlash_model=sdl.enum.backlashModel.Off  backlash_distance=1e-3 mm  x0=0 mm  r_base=0.1 m  hardstop_model=simscape.enum.hardstop.smooth  transition=1e-4 mm  backlash_stiffness=1e7 N/m  backlash_damping=1e6 N*s/m  e=0  v_tol=0.001 m/s  mu_visc=[ 0 0 ] N*m/(rad/s)  enable_faults=simscape.enum.onoff.off  efficiency_fault=0.05  external_fault=simscape.enum.onoff.off  temporal_fault=simscape.enum.onoff.off  fault_time=5 s  fault_angles=pi / 12 rad  report_fault=(1)-1  thermal_mass=50 J/K  temperature_specify=off  temperature_priority=High  temperature=300 K  temperature_nominal_specify=off  temperature_nominal_unit=K  temperature_nominal_value=1  x_backlash_specify=off  x_backlash_priority=None  x_backlash=0 mm  x_backlash_nominal_specify=off  x_backlash_nominal_unit=mm  x_backlash_nominal_value=1  f_hardstop_specify=off  f_hardstop_priority=None  f_hardstop=0 N  f_hardstop_nominal_specify=off  f_hardstop_nominal_unit=N  f_hardstop_nominal_value=1  v_backlash_specify=off  v_backlash_priority=None  v_backlash=0 m/s  v_backlash_nominal_specify=off  v_backlash_nominal_unit=m/s  v_backlash_nominal_value=1
  D : PMIOPort  Side=Left
  S1 : PMIOPort  Port=2  Side=Right
  S2 : PMIOPort  Port=3  Side=Right
  connections:
  D/RConn1 -- Input Pinion Crown Gear/LConn1
  Input Pinion Crown Gear/RConn1 -- Sun-Planet Worm Gear 2/LConn1 -- Sun-Planet Worm Gear 1/LConn1
  Worm Wheels/RConn1 -- Sun-Planet Worm Gear 2/RConn1
  S1/RConn1 -- Sun-Planet Worm Gear 1/RConn2
  S2/RConn1 -- Sun-Planet Worm Gear 2/RConn2
  Sun-Planet Worm Gear 1/RConn1 -- Worm Wheels/LConn1

== system sdl_testbed/Front Tires/Subsystem ==
  In1 : Inport
  Simulink-PS Converter : nesl_utility/Simulink-PS Converter  PhysicalDomain=network_engine_domain  SubClassName=ps_input  LeftPortType=input  RightPortType=output  PseudoPeriodic=off  Frequencies=[]  NoiseDistribution=none  NoiseParameters=[]  Unit=1  AffineConversion=off  FilteringAndDerivatives=zero  SimscapeFilterOrder=1  InputFilterTimeConstant=0.001  UdotUserProvided=1
  Conn1 : PMIOPort  Side=Right
  wires:
  In1/1 -> Simulink-PS Converter/1
  connections:
  Simulink-PS Converter/RConn1 -- Conn1/RConn1

== system sdl_testbed/Front Tires/Subsystem1 ==
  In1 : Inport
  Simulink-PS Converter : nesl_utility/Simulink-PS Converter  PhysicalDomain=network_engine_domain  SubClassName=ps_input  LeftPortType=input  RightPortType=output  PseudoPeriodic=off  Frequencies=[]  NoiseDistribution=none  NoiseParameters=[]  Unit=1  AffineConversion=off  FilteringAndDerivatives=zero  SimscapeFilterOrder=1  InputFilterTimeConstant=0.001  UdotUserProvided=1
  Conn1 : PMIOPort  Side=Right
  wires:
  In1/1 -> Simulink-PS Converter/1
  connections:
  Simulink-PS Converter/RConn1 -- Conn1/RConn1

== system sdl_testbed/Rear Differential/Open ==
  Differential : sdl_lib/Gears/Differential  driveshaft_location=2  cd_ratio=1.33  friction_model=1  efficiency=[ 0.9 0.92 ]  temperature_TLU=[ 280 300 320 ] K  efficiency_ss_TLU=[ 0.95 0.9 0.85 ]  efficiency_cd_TLU=[ 0.95 0.9 0.85 ]  pwr_thr=[ 0.001 0.001 ] W  mu_visc=[ 0 0 ] N*m/(rad/s)  model_inertia=0  carrier_inertia=0.001 kg*m^2  planet_inertia=0.001 kg*m^2  thermal_mass=50 J/K  T_init=300 K
  D : PMIOPort  Side=Left
  S1 : PMIOPort  Port=2  Side=Right
  S2 : PMIOPort  Port=3  Side=Right
  connections:
  D/RConn1 -- Differential/LConn1
  S1/RConn1 -- Differential/RConn1
  S2/RConn1 -- Differential/RConn2

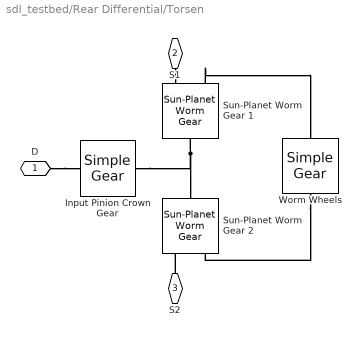
== system sdl_testbed/Rear Differential/Torsen ==
  Input Pinion Crown Gear : sdl_lib/Gears/Simple Gear  ratio=2  rotation_direction=3-2*(1)  friction_model=1  T_noload=0.1 N*m  T_nom=5 N*m  efficiency_nom=0.8  efficiency=0.92  temperature_TLU=[ 280 300 320 ] K  load_TLU=[ 1 5 10 ] N*m  efficiency_TLU=[ 0.95 0.9 0.85 ]  efficiency_TLU2=[ 0.85 0.8 0.75; 0.95 0.9 0.85; 0.85 0.8 0.7 ]  w_thr=0.01 rad/s  pwr_thr=0.001 W  backlash_model=sdl.enum.backlashModel.Off  backlash_distance=1e-3 mm  x0=0 mm  r_base=0.1 m  hardstop_model=simscape.enum.hardstop.smooth  transition=1e-4 mm  backlash_stiffness=1e7 N/m  backlash_damping=1e6 N*s/m  e=0  v_tol=0.001 m/s  mu_visc=[ 0 0 ] N*m/(rad/s)  enable_faults=simscape.enum.onoff.off  efficiency_fault=0.05  external_fault=simscape.enum.onoff.off  temporal_fault=simscape.enum.onoff.off  fault_time=5 s  fault_angles=pi / 12 rad  report_fault=(1)-1  thermal_mass=50 J/K  temperature_specify=off  temperature_priority=High  temperature=300 K  temperature_nominal_specify=off  temperature_nominal_unit=K  temperature_nominal_value=1  x_backlash_specify=off  x_backlash_priority=None  x_backlash=0 mm  x_backlash_nominal_specify=off  x_backlash_nominal_unit=mm  x_backlash_nominal_value=1  f_hardstop_specify=off  f_hardstop_priority=None  f_hardstop=0 N  f_hardstop_nominal_specify=off  f_hardstop_nominal_unit=N  f_hardstop_nominal_value=1  v_backlash_specify=off  v_backlash_priority=None  v_backlash=0 m/s  v_backlash_nominal_specify=off  v_backlash_nominal_unit=m/s  v_backlash_nominal_value=1
  Sun-Planet Worm Gear 1 : sdl_lib/Gears/Planetary Subcomponents/Sun-Planet Worm Gear  ratio=2  thread_type=1  friction_model=2  friction_parameterization=2  pr_ang=17.5 deg  lead_ang=20 deg  fr_coeff=0.08  eff_wg=0.74  eff_gw=-0.1  temperature_TLU=[ 280 300 320 ] K  efficiency_wg_TLU=[ 0.75 0.7 0.65 ]  efficiency_gw_TLU=[ 0.5 0.45 0.4 ]  pwr_thr=0.001 W  mu_visc=[ 0 0 ] N*m/(rad/s)  thermal_mass=50 J/K  temperature_specify=off  temperature_priority=High  temperature=300 K  temperature_nominal_specify=off  temperature_nominal_unit=K  temperature_nominal_value=1
      settings: InternalSimscapePortConfiguration="{\"Bottom\":[],\"Left\":[{\"id\":\"C\",\"label\":\"C\",\"type\":\"foundation.mechanical.rotational.rotational\"}],\"Right\":[{\"id\":\"W\",\"label\":\"W\",\"type\":\"foundation.mechanical.rotational.rotational\"},{\"id\":\"S\",\"label\":\"S\",\"type\":\"foundation.mechanical.rotational.rotational\"}],\"Top\":[]}"
  Sun-Planet Worm Gear 2 : sdl_lib/Gears/Planetary Subcomponents/Sun-Planet Worm Gear  ratio=2  thread_type=1  friction_model=2  friction_parameterization=2  pr_ang=17.5 deg  lead_ang=20 deg  fr_coeff=0.08  eff_wg=0.74  eff_gw=-0.1  temperature_TLU=[ 280 300 320 ] K  efficiency_wg_TLU=[ 0.75 0.7 0.65 ]  efficiency_gw_TLU=[ 0.5 0.45 0.4 ]  pwr_thr=0.001 W  mu_visc=[ 0 0 ] N*m/(rad/s)  thermal_mass=50 J/K  temperature_specify=off  temperature_priority=High  temperature=300 K  temperature_nominal_specify=off  temperature_nominal_unit=K  temperature_nominal_value=1
      settings: InternalSimscapePortConfiguration="{\"Bottom\":[],\"Left\":[{\"id\":\"C\",\"label\":\"C\",\"type\":\"foundation.mechanical.rotational.rotational\"}],\"Right\":[{\"id\":\"W\",\"label\":\"W\",\"type\":\"foundation.mechanical.rotational.rotational\"},{\"id\":\"S\",\"label\":\"S\",\"type\":\"foundation.mechanical.rotational.rotational\"}],\"Top\":[]}"
  Worm Wheels : sdl_lib/Gears/Simple Gear  ratio=1  rotation_direction=3-2*(2)  friction_model=1  T_noload=0.1 N*m  T_nom=5 N*m  efficiency_nom=0.8  efficiency=0.92  temperature_TLU=[ 280 300 320 ] K  load_TLU=[ 1 5 10 ] N*m  efficiency_TLU=[ 0.95 0.9 0.85 ]  efficiency_TLU2=[ 0.85 0.8 0.75; 0.95 0.9 0.85; 0.85 0.8 0.7 ]  w_thr=0.01 rad/s  pwr_thr=0.001 W  backlash_model=sdl.enum.backlashModel.Off  backlash_distance=1e-3 mm  x0=0 mm  r_base=0.1 m  hardstop_model=simscape.enum.hardstop.smooth  transition=1e-4 mm  backlash_stiffness=1e7 N/m  backlash_damping=1e6 N*s/m  e=0  v_tol=0.001 m/s  mu_visc=[ 0 0 ] N*m/(rad/s)  enable_faults=simscape.enum.onoff.off  efficiency_fault=0.05  external_fault=simscape.enum.onoff.off  temporal_fault=simscape.enum.onoff.off  fault_time=5 s  fault_angles=pi / 12 rad  report_fault=(1)-1  thermal_mass=50 J/K  temperature_specify=off  temperature_priority=High  temperature=300 K  temperature_nominal_specify=off  temperature_nominal_unit=K  temperature_nominal_value=1  x_backlash_specify=off  x_backlash_priority=None  x_backlash=0 mm  x_backlash_nominal_specify=off  x_backlash_nominal_unit=mm  x_backlash_nominal_value=1  f_hardstop_specify=off  f_hardstop_priority=None  f_hardstop=0 N  f_hardstop_nominal_specify=off  f_hardstop_nominal_unit=N  f_hardstop_nominal_value=1  v_backlash_specify=off  v_backlash_priority=None  v_backlash=0 m/s  v_backlash_nominal_specify=off  v_backlash_nominal_unit=m/s  v_backlash_nominal_value=1
  D : PMIOPort  Side=Left
  S1 : PMIOPort  Port=2  Side=Right
  S2 : PMIOPort  Port=3  Side=Right
  connections:
  Sun-Planet Worm Gear 1/LConn1 -- Input Pinion Crown Gear/RConn1 -- Sun-Planet Worm Gear 2/LConn1
  S2/RConn1 -- Sun-Planet Worm Gear 2/RConn2
  Sun-Planet Worm Gear 1/RConn1 -- Worm Wheels/LConn1
  D/RConn1 -- Input Pinion Crown Gear/LConn1
  S1/RConn1 -- Sun-Planet Worm Gear 1/RConn2
  Worm Wheels/RConn1 -- Sun-Planet Worm Gear 2/RConn1

== system sdl_testbed/Rear Tires/Subsystem ==
  In1 : Inport
  Simulink-PS Converter : nesl_utility/Simulink-PS Converter  PhysicalDomain=network_engine_domain  SubClassName=ps_input  LeftPortType=input  RightPortType=output  PseudoPeriodic=off  Frequencies=[]  NoiseDistribution=none  NoiseParameters=[]  Unit=1  AffineConversion=off  FilteringAndDerivatives=zero  SimscapeFilterOrder=1  InputFilterTimeConstant=0.001  UdotUserProvided=1
  Conn1 : PMIOPort  Side=Right
  wires:
  In1/1 -> Simulink-PS Converter/1
  connections:
  Simulink-PS Converter/RConn1 -- Conn1/RConn1

== system sdl_testbed/Rear Tires/Subsystem1 ==
  In1 : Inport
  Simulink-PS Converter : nesl_utility/Simulink-PS Converter  PhysicalDomain=network_engine_domain  SubClassName=ps_input  LeftPortType=input  RightPortType=output  PseudoPeriodic=off  Frequencies=[]  NoiseDistribution=none  NoiseParameters=[]  Unit=1  AffineConversion=off  FilteringAndDerivatives=zero  SimscapeFilterOrder=1  InputFilterTimeConstant=0.001  UdotUserProvided=1
  Conn1 : PMIOPort  Side=Right
  wires:
  In1/1 -> Simulink-PS Converter/1
  connections:
  Simulink-PS Converter/RConn1 -- Conn1/RConn1

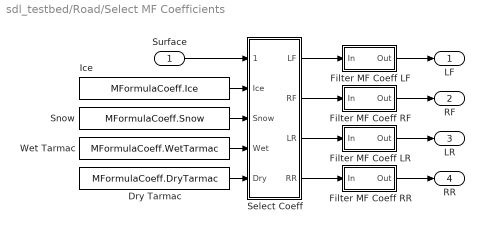
== system sdl_testbed/Road/Select MF Coefficients ==
  Surface : Inport
  Dry Tarmac : Constant  Value=MFormulaCoeff.DryTarmac  SampleTime=0
  Filter MF Coeff LF : Subsystem  mask(First-order lag supporting vector signals){b=0.01, x_initial=MFormulaCoeff.DryTarmac}
      mask prompts: b "Filter time constant"; x_initial "Initial output"
      mask help: Models a lag of the form 1/(b*s+1) where s is the Laplace operator.
  Filter MF Coeff LR : Subsystem  mask(First-order lag supporting vector signals){b=0.01, x_initial=MFormulaCoeff.DryTarmac}
      mask prompts: b "Filter time constant"; x_initial "Initial output"
      mask help: Models a lag of the form 1/(b*s+1) where s is the Laplace operator.
  Filter MF Coeff RF : Subsystem  mask(First-order lag supporting vector signals){b=0.01, x_initial=MFormulaCoeff.DryTarmac}
      mask prompts: b "Filter time constant"; x_initial "Initial output"
      mask help: Models a lag of the form 1/(b*s+1) where s is the Laplace operator.
  Filter MF Coeff RR : Subsystem  mask(First-order lag supporting vector signals){b=0.01, x_initial=MFormulaCoeff.DryTarmac}
      mask prompts: b "Filter time constant"; x_initial "Initial output"
      mask help: Models a lag of the form 1/(b*s+1) where s is the Laplace operator.
  Ice : Constant  Value=MFormulaCoeff.Ice  SampleTime=0
  Select Coeff : Subsystem
  Snow : Constant  Value=MFormulaCoeff.Snow  SampleTime=0
  Wet Tarmac : Constant  Value=MFormulaCoeff.WetTarmac  SampleTime=0
  LF : Outport  VectorParamsAs1DForOutWhenUnconnected=off
  RF : Outport  Port=2  VectorParamsAs1DForOutWhenUnconnected=off
  LR : Outport  Port=3  VectorParamsAs1DForOutWhenUnconnected=off
  RR : Outport  Port=4  VectorParamsAs1DForOutWhenUnconnected=off
  wires:
  Select Coeff/2(RF) -> Filter MF Coeff RF/1(In)
  Select Coeff/1(LF) -> Filter MF Coeff LF/1(In)
  Select Coeff/4(RR) -> Filter MF Coeff RR/1(In)
  Select Coeff/3(LR) -> Filter MF Coeff LR/1(In)
  Surface/1 -> Select Coeff/1(Surface)
  Snow/1 -> Select Coeff/3(Snow)
  Wet Tarmac/1 -> Select Coeff/4(Wet)
  Ice/1 -> Select Coeff/2(Ice)
  Dry Tarmac/1 -> Select Coeff/5(Dry)
  Filter MF Coeff LF/1(Out) -> LF/1
  Filter MF Coeff RF/1(Out) -> RF/1
  Filter MF Coeff LR/1(Out) -> LR/1
  Filter MF Coeff RR/1(Out) -> RR/1
